simulink model "prob2"  (R2020b)
settings: Solver=FixedStepDiscrete  StartTime=0.0  StopTime=150  FixedStep=1  RelTol=1e-3  EnableMultiTasking=on
libraries: simulink x1
settings Model: Creator=nadee  LastModifiedBy=nadee

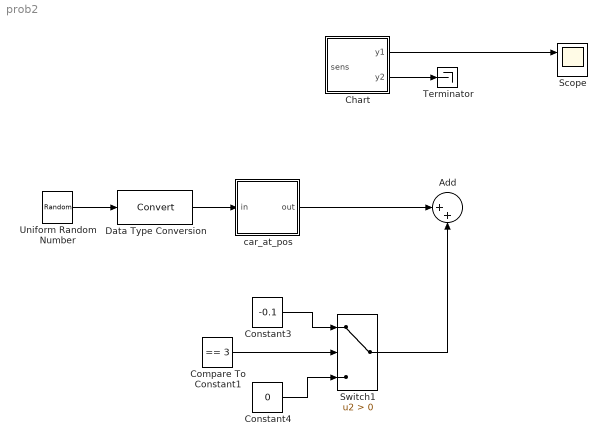
== system prob2 ==
  Add : Sum  Inputs=|++
  Chart : Stateflow chart  TreatAsAtomicUnit=on
  Compare To Constant1 : simulink/Logic and Bit Operations/Compare To Constant  relop===  const=3  OutDataTypeStr=boolean  ZeroCross=off
  Constant3 : Constant  Value=-0.1
  Constant4 : Constant  Value=0
  Data Type Conversion : DataTypeConversion
  Scope : Scope  NumInputPorts=2
  Switch1 : Switch  Criteria=u2 > Threshold
  Terminator : Terminator
  Uniform Random Number : UniformRandomNumber  Minimum=0  Maximum=100  Seed=177836  SampleTime=0
  car_at_pos : Stateflow chart  TreatAsAtomicUnit=on
  wires:
  Chart/2(y2) -> Terminator/1
  Chart/1(y1) -> Scope/1
  Uniform Random Number/1 -> Data Type Conversion/1
  Data Type Conversion/1 -> car_at_pos/1(in)
  Constant3/1 -> Switch1/1
  Compare To Constant1/1 -> Switch1/2
  Constant4/1 -> Switch1/3
  car_at_pos/1(out) -> Add/1
  Switch1/1 -> Add/2

== stateflow chart prob2/car_at_pos ==
  (default) -> (junction 1) : {out = in >98;}
  data: out output; in input

== stateflow chart prob2/Chart ==
  state Stop
    y1 = RED;
    y2 = GREEN;
  state StopForTraffic
    y1 = RED;
    y2 =  GREEN;
  state StopToGo
    y1 = RED;
    y2 = YELLOW;
  state GoToStop
    y1 = YELLOW;
    y2 = RED;
  state Go
    y1 = GREEN;
    y2 = RED;
  (default) -> Stop
  Stop -> StopForTraffic : after(20,tick)
  StopForTraffic -> StopToGo : [sens]
  GoToStop -> Stop : after(3,tick)
  StopToGo -> Go : after(3,tick)
  Go -> GoToStop : after(10,tick)
  data: sens input; y1 output; y2 output; RED constant double =1; YELLOW constant double =2; GREEN constant double =3
